simulink model "Ray_tracing_hit"  (R2025b)
settings: Solver=FixedStepAuto  StartTime=0.0  StopTime=10.0  RelTol=1e-3
undefined symbols (not defined in the file): d_raycount, sal_atmos_coef, t_reflect, t_size
settings Model: DataDictionary=Ray_tracing_hit_data.sldd  Creator=mauro  LastModifiedBy=mauro

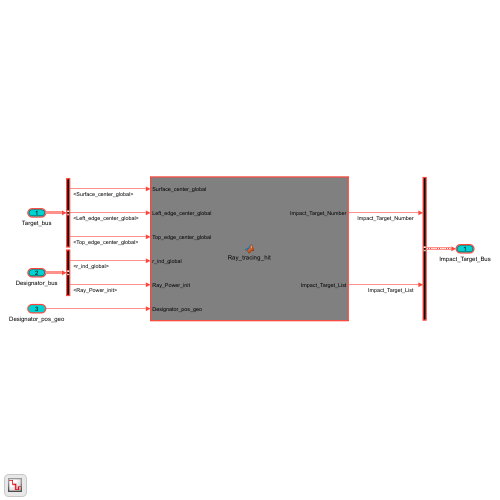
[thumbnail: Simulink's stored preview of the top-level diagram]
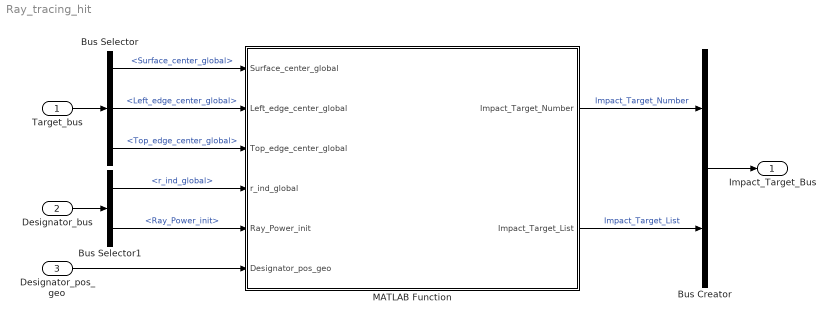
== system Ray_tracing_hit ==
  Target_bus : Inport  OutDataTypeStr=Bus: Target_bus
  Designator_bus : Inport  Port=2  OutDataTypeStr=Bus: Designator_bus
  Designator_pos_geo : Inport  Port=3  PortDimensions=[3 1]
  Bus Creator : BusCreator  Inputs=2  OutDataTypeStr=Bus: Impact_Target_Bus  NonVirtualBus=on
  Bus Selector : BusSelector  OutputSignals=Surface_center_global,Left_edge_center_global,Top_edge_center_global
  Bus Selector1 : BusSelector  OutputSignals=r_ind_global,Ray_Power_init
  MATLAB Function : MATLAB Function  TreatAsAtomicUnit=on
  Impact_Target_Bus : Outport  OutDataTypeStr=Bus: Impact_Target_Bus  BusOutputAsStruct=on
  wires:
  Designator_pos_geo/1 -> MATLAB Function/6(Designator_pos_geo)
  MATLAB Function/2(Impact_Target_List) -> Bus Creator/2  "Impact_Target_List"
  MATLAB Function/1(Impact_Target_Number) -> Bus Creator/1  "Impact_Target_Number"
  Bus Creator/1 -> Impact_Target_Bus/1
  Target_bus/1 -> Bus Selector/1
  Designator_bus/1 -> Bus Selector1/1
  Bus Selector/1 -> MATLAB Function/1(Surface_center_global)  "<Surface_center_global>"
  Bus Selector/2 -> MATLAB Function/2(Left_edge_center_global)  "<Left_edge_center_global>"
  Bus Selector/3 -> MATLAB Function/3(Top_edge_center_global)  "<Top_edge_center_global>"
  Bus Selector1/1 -> MATLAB Function/4(r_ind_global)  "<r_ind_global>"
  Bus Selector1/2 -> MATLAB Function/5(Ray_Power_init)  "<Ray_Power_init>"

== matlab function Ray_tracing_hit/MATLAB Function ==
  settings: updateMethod=DISCRETE
  data: Impact_Target_Number output; Surface_center_global input; Impact_Target_List output; Left_edge_center_global input; Top_edge_center_global input; r_ind_global input; Ray_Power_init input; Designator_pos_geo input; d_raycount parameter; sal_atmos_coef parameter; t_size parameter; t_reflect parameter
function [Impact_Target_Number,Impact_Target_List] = Ray_tracing_hit(Surface_center_global,Left_edge_center_global,Top_edge_center_global,r_ind_global,Ray_Power_init,Designator_pos_geo,d_raycount,sal_atmos_coef,t_size, t_reflect)

    Ray_tracing_data     = zeros(3,length(Surface_center_global));
    Impact_Target_Number = 0;
    Impact_Target_List   = zeros(5,d_raycount);
    % Each column of Impact_Target_List contains the data of 1 ray of the
    % laser pulse. The first row shows total distance from the designator
    % to the target, the second and third row shows distance from the
    % surface center to impact point in local reference system (the
    % direction may vary depending on the surface), the fourth row shows
    % the surface code number that received impact, and the fifth row shows
    % the power carried by the ray.

    for i = 1:d_raycount
    
        for j = 1:length(Surface_center_global)
    
            [t,u,v]                 = Ray_tracing(Surface_center_global(:, j), Left_edge_center_global(:, j), Top_edge_center_global(:, j), r_ind_global(:, i), Designator_pos_geo);
            Ray_tracing_data(1:3,j) = [t,u,v]';
    
        if j==1 || j==2
    
            if abs(u)>=t_size(2)/2 || abs(v)>=t_size(3)/2
    
                Ray_tracing_data(:,j)=zeros(3,1);
    
            end
    
        elseif j==3 || j==4
    
            if abs(u)>=t_size(1)/2 || abs(v)>=t_size(3)/2
    
                Ray_tracing_data(:,j)=zeros(3,1);
    
            end
    
        else    
    
            if abs(u)>=t_size(2)/2 || abs(v)>=t_size(1)/2
    
                Ray_tracing_data(:,j)=zeros(3,1);
    
            end
    
        end
    
        end
    
        t               = Ray_tracing_data(1,:);
        Possible_impact = find(t~=0);
    
        if isempty(Possible_impact)
    
            Impact_Target_Number = Impact_Target_Number+0;
    
        else
    
            [~,x]                       = min(abs(t(Possible_impact)));
            Impact_Target_Number        = Impact_Target_Number+1;
            Impact_Target_Surface       = Possible_impact(x);
            Impact_Target_Data          = Ray_tracing_data(:,Impact_Target_Surface);
    
            Impact_Target_List(1:3,Impact_Target_Number)    = Impact_Target_Data;
            Impact_Target_List(4,Impact_Target_Number)      = Impact_Target_Surface;
            Impact_Target_List(5,Impact_Target_Number)      = Ray_Power_init*exp(-sal_atmos_coef*Impact_Target_List(1,Impact_Target_Number))*t_reflect(Impact_Target_List(4,Impact_Target_Number));
      
        end
        
    end
    
end
